simulink model "findClosestPathParameter_th"  (R2020a)
settings: Solver=VariableStepAuto  StartTime=0.0  StopTime=10.0  RelTol=1e-3
undefined symbols (not defined in the file or in its folder): initPathParam, kitePos, pathElev, pathHeight, pathWidth
libraries: findClosestPathParameter_ul x1
settings Model: Creator=Ayaz  LastModifiedBy=Ayaz

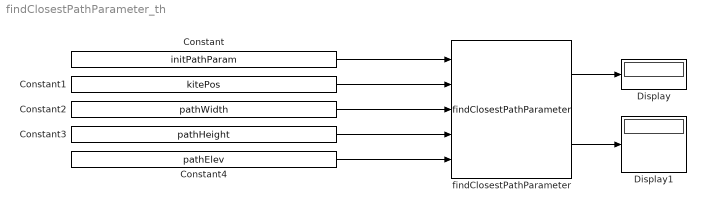
== system findClosestPathParameter_th ==
  Constant : Constant  Value=initPathParam
  Constant1 : Constant  Value=kitePos
  Constant2 : Constant  Value=pathWidth
  Constant3 : Constant  Value=pathHeight
  Constant4 : Constant  Value=pathElev
  Display : Display
  Display1 : Display
  findClosestPathParameter : findClosestPathParameter_ul/findClosestPathParameter  SystemSampleTime=-1  Latency=0  AutoFrameSizeCalculation=off
  wires:
  Constant/1 -> findClosestPathParameter/1
  Constant1/1 -> findClosestPathParameter/2
  Constant2/1 -> findClosestPathParameter/3
  Constant3/1 -> findClosestPathParameter/4
  Constant4/1 -> findClosestPathParameter/5
  findClosestPathParameter/1 -> Display/1
  findClosestPathParameter/2 -> Display1/1
